simulink model "Electrical787"  (R2013a)
settings: Solver=ode45  StartTime=0.0  StopTime=MSSN.gen.time(end)  RelTol=1e-3
InitFcn:
  | load('SampleOutput.mat')
  | 
  | load('SampleFuelBurn.mat')
undefined symbols (not defined in the file): ailerons, B_737, elevator, FuelBurn, landing_gear, rudder, thrust_rev
libraries: PowerFlowLib x95, simulink x17
(part 16 of 17)

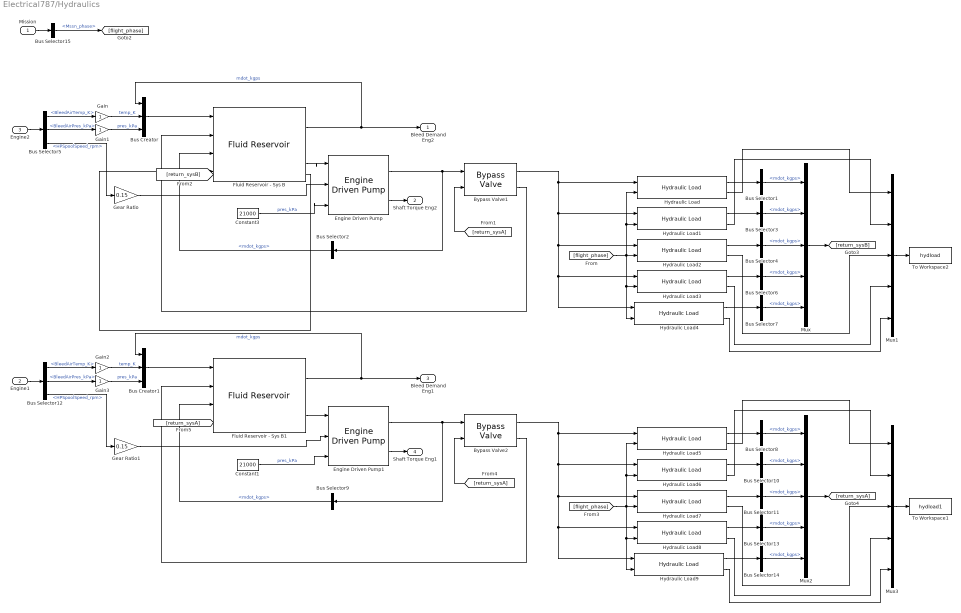
== system Electrical787/Hydraulics  ==
  Mission : Inport
  Engine1 : Inport  Port=2
  Engine2 : Inport  Port=3
  Bus Creator : BusCreator  Inputs=3
  Bus Creator1 : BusCreator  Inputs=3
  Bus Selector{1..4,6..11,13..14} (12 alike) : BusSelector  OutputSignals=mdot_kgps
  Bus Selector12 : BusSelector  OutputSignals=Bleed.BleedAirTemp_K,Bleed.BleedAirPres_kPa,Spools.HPSpoolSpeed_rpm
  Bus Selector15 : BusSelector  OutputSignals=Mssn_phase
  Bus Selector5 : BusSelector  OutputSignals=Bleed.BleedAirTemp_K,Bleed.BleedAirPres_kPa,Spools.HPSpoolSpeed_rpm
  Bypass Valve1 : PowerFlowLib/Energy & Power Systems/Hydraulic/Bypass Valve
  Bypass Valve2 : PowerFlowLib/Energy & Power Systems/Hydraulic/Bypass Valve
  Constant1 : Constant  Value=21000
  Constant3 : Constant  Value=21000
  Engine Driven Pump : PowerFlowLib/Energy & Power Systems/Hydraulic/Engine Driven Pump  RPM=3750  disp=39  eta_mech=95  eta_v=85  nom_T=40  nom_w=393  nom_delP=20684
  Engine Driven Pump1 : PowerFlowLib/Energy & Power Systems/Hydraulic/Engine Driven Pump  RPM=3750  disp=39  eta_mech=95  eta_v=85  nom_T=40  nom_w=393  nom_delP=20684
  Fluid Reservoir - Sys B : PowerFlowLib/Energy & Power Systems/Hydraulic/Fluid Reservoir  res_vol=.25  bleed_flowrate=.05  pres_loss=1  T_init=300  P_init=1500  mass_init=30
  Fluid Reservoir - Sys B1 : PowerFlowLib/Energy & Power Systems/Hydraulic/Fluid Reservoir  res_vol=.25  bleed_flowrate=.05  pres_loss=1  T_init=300  P_init=1500  mass_init=30
  Gain{,1..3} (4 alike) : Gain
  Gear Ratio : Gain  Gain=0.15
  Gear Ratio1 : Gain  Gain=0.15
  Hydraulic Load : PowerFlowLib/Energy & Power Systems/Hydraulic/Hydraulic Load  fileslct=off  filename=HydraulicLoad.mat  filedir=C:\Users\mwillms4\Dropbox\School\Graduate\Research\PowerFlow Development\PowerFlow Summer 2013\PropertyTables\HydraulicLoad.mat  var_struct=HydraulicLoad  h_load=B_737 - rudder
  Hydraulic Load1 : PowerFlowLib/Energy & Power Systems/Hydraulic/Hydraulic Load  fileslct=off  filename=HydraulicLoad.mat  filedir=C:\Users\mwillms4\Dropbox\School\Graduate\Research\PowerFlow Development\PowerFlow Summer 2013\PropertyTables\HydraulicLoad.mat  var_struct=HydraulicLoad  h_load=B_737 - ailerons
  Hydraulic Load2 : PowerFlowLib/Energy & Power Systems/Hydraulic/Hydraulic Load  fileslct=off  filename=HydraulicLoad.mat  filedir=C:\Users\mwillms4\Dropbox\School\Graduate\Research\PowerFlow Development\PowerFlow Summer 2013\PropertyTables\HydraulicLoad.mat  var_struct=HydraulicLoad  h_load=B_737 - elevator
  Hydraulic Load3 : PowerFlowLib/Energy & Power Systems/Hydraulic/Hydraulic Load  fileslct=off  filename=HydraulicLoad.mat  filedir=C:\Users\mwillms4\Dropbox\School\Graduate\Research\PowerFlow Development\PowerFlow Summer 2013\PropertyTables\HydraulicLoad.mat  var_struct=HydraulicLoad  h_load=B_737 - landing_gear
  Hydraulic Load4 : PowerFlowLib/Energy & Power Systems/Hydraulic/Hydraulic Load  fileslct=off  filename=HydraulicLoad.mat  filedir=C:\Users\mwillms4\Dropbox\School\Graduate\Research\PowerFlow Development\PowerFlow Summer 2013\PropertyTables\HydraulicLoad.mat  var_struct=HydraulicLoad  h_load=B_737 - thrust_rev
  Hydraulic Load5 : PowerFlowLib/Energy & Power Systems/Hydraulic/Hydraulic Load  fileslct=off  filename=HydraulicLoad.mat  filedir=C:\Users\mwillms4\Dropbox\School\Graduate\Research\PowerFlow Development\PowerFlow Summer 2013\PropertyTables\HydraulicLoad.mat  var_struct=HydraulicLoad  h_load=B_737 - rudder
  Hydraulic Load6 : PowerFlowLib/Energy & Power Systems/Hydraulic/Hydraulic Load  fileslct=off  filename=HydraulicLoad.mat  filedir=C:\Users\mwillms4\Dropbox\School\Graduate\Research\PowerFlow Development\PowerFlow Summer 2013\PropertyTables\HydraulicLoad.mat  var_struct=HydraulicLoad  h_load=B_737 - ailerons
  Hydraulic Load7 : PowerFlowLib/Energy & Power Systems/Hydraulic/Hydraulic Load  fileslct=off  filename=HydraulicLoad.mat  filedir=C:\Users\mwillms4\Dropbox\School\Graduate\Research\PowerFlow Development\PowerFlow Summer 2013\PropertyTables\HydraulicLoad.mat  var_struct=HydraulicLoad  h_load=B_737 - elevator
  Hydraulic Load8 : PowerFlowLib/Energy & Power Systems/Hydraulic/Hydraulic Load  fileslct=off  filename=HydraulicLoad.mat  filedir=C:\Users\mwillms4\Dropbox\School\Graduate\Research\PowerFlow Development\PowerFlow Summer 2013\PropertyTables\HydraulicLoad.mat  var_struct=HydraulicLoad  h_load=B_737 - landing_gear
  Hydraulic Load9 : PowerFlowLib/Energy & Power Systems/Hydraulic/Hydraulic Load  fileslct=off  filename=HydraulicLoad.mat  filedir=C:\Users\mwillms4\Dropbox\School\Graduate\Research\PowerFlow Development\PowerFlow Summer 2013\PropertyTables\HydraulicLoad.mat  var_struct=HydraulicLoad  h_load=B_737 - thrust_rev
  Mux{,1..3} (4 alike) : Mux  Inputs=5
  To Workspace1 : ToWorkspace  VariableName=hydload1  SampleTime=10  SaveFormat=Structure With Time
  To Workspace2 : ToWorkspace  VariableName=hydload  SampleTime=10  SaveFormat=Structure With Time
  Bleed Demand Eng2 : Outport
  Shaft Torque Eng2 : Outport  Port=2
  Bleed Demand Eng1 : Outport  Port=3
  Shaft Torque Eng1 : Outport  Port=4
  wires:
  Bus Creator/1 -> Fluid Reservoir - Sys B/1
  Bus Selector5/1 -> Gain/1  "<BleedAirTemp_K>"
  Bus Selector5/2 -> Gain1/1  "<BleedAirPres_kPa>"
  Hydraulic Load/1 -> Bus Selector1/1
  Fluid Reservoir - Sys B/2 -> Engine Driven Pump/1
  Engine Driven Pump/1 -> Bypass Valve1/1, Bus Selector2/1
  Bypass Valve1/1 -> Hydraulic Load3/1, Hydraulic Load4/1, Hydraulic Load2/1, Hydraulic Load1/1, Hydraulic Load/1
  Gear Ratio/1 -> Engine Driven Pump/2
  Bus Selector2/1 -> Fluid Reservoir - Sys B/3  "<mdot_kgps>"
  Bypass Valve1/2 -> Fluid Reservoir - Sys B/2
  Fluid Reservoir - Sys B/1 -> Bus Creator/1, Bleed Demand Eng2/1  "mdot_kgps"
  Hydraulic Load1/2 -> Mux1/2
  Hydraulic Load2/2 -> Mux1/3
  Hydraulic Load1/1 -> Bus Selector3/1
  Hydraulic Load2/1 -> Bus Selector4/1
  Bus Selector3/1 -> Mux/2  "<mdot_kgps>"
  Bus Selector1/1 -> Mux/1  "<mdot_kgps>"
  Bus Selector4/1 -> Mux/3  "<mdot_kgps>"
  Mux/1 -> [return_sysB]
  [return_sysA] -> Bypass Valve1/2
  [return_sysB] -> Fluid Reservoir - Sys B/4
  [flight_phase] -> Hydraulic Load/2, Hydraulic Load1/2, Hydraulic Load3/2, Hydraulic Load4/2, Hydraulic Load2/2
  Engine2/1 -> Bus Selector5/1
  Hydraulic Load3/1 -> Bus Selector6/1
  Hydraulic Load4/1 -> Bus Selector7/1
  Hydraulic Load4/2 -> Mux1/5
  Hydraulic Load3/2 -> Mux1/4
  Bus Selector6/1 -> Mux/4  "<mdot_kgps>"
  Bus Selector7/1 -> Mux/5  "<mdot_kgps>"
  Mission/1 -> Bus Selector15/1
  Bus Selector15/1 -> [flight_phase]  "<Mssn_phase>"
  Gain/1 -> Bus Creator/2  "temp_K"
  Gain1/1 -> Bus Creator/3  "pres_kPa"
  Constant3/1 -> Engine Driven Pump/3  "pres_kPa"
  Hydraulic Load/2 -> Mux1/1
  Bus Selector5/3 -> Gear Ratio/1  "<HPSpoolSpeed_rpm>"
  Engine Driven Pump/2 -> Shaft Torque Eng2/1
  Mux1/1 -> To Workspace2/1
  Bus Creator1/1 -> Fluid Reservoir - Sys B1/1
  Bus Selector12/1 -> Gain2/1  "<BleedAirTemp_K>"
  Bus Selector12/2 -> Gain3/1  "<BleedAirPres_kPa>"
  Hydraulic Load5/1 -> Bus Selector8/1
  Fluid Reservoir - Sys B1/2 -> Engine Driven Pump1/1
  Engine Driven Pump1/1 -> Bus Selector9/1, Bypass Valve2/1
  Bypass Valve2/1 -> Hydraulic Load8/1, Hydraulic Load9/1, Hydraulic Load7/1, Hydraulic Load6/1, Hydraulic Load5/1
  Gear Ratio1/1 -> Engine Driven Pump1/2
  Bus Selector9/1 -> Fluid Reservoir - Sys B1/3  "<mdot_kgps>"
  Bypass Valve2/2 -> Fluid Reservoir - Sys B1/2
  Fluid Reservoir - Sys B1/1 -> Bus Creator1/1, Bleed Demand Eng1/1  "mdot_kgps"
  Hydraulic Load6/2 -> Mux3/2
  Hydraulic Load7/2 -> Mux3/3
  Hydraulic Load6/1 -> Bus Selector10/1
  Hydraulic Load7/1 -> Bus Selector11/1
  Bus Selector10/1 -> Mux2/2  "<mdot_kgps>"
  Bus Selector8/1 -> Mux2/1  "<mdot_kgps>"
  Bus Selector11/1 -> Mux2/3  "<mdot_kgps>"
  Mux2/1 -> [return_sysA]
  [return_sysA] -> Bypass Valve2/2
  [return_sysA] -> Fluid Reservoir - Sys B1/4
  [flight_phase] -> Hydraulic Load5/2, Hydraulic Load6/2, Hydraulic Load8/2, Hydraulic Load9/2, Hydraulic Load7/2
  Engine1/1 -> Bus Selector12/1
  Hydraulic Load8/1 -> Bus Selector13/1
  Hydraulic Load9/1 -> Bus Selector14/1
  Hydraulic Load9/2 -> Mux3/5
  Hydraulic Load8/2 -> Mux3/4
  Bus Selector13/1 -> Mux2/4  "<mdot_kgps>"
  Bus Selector14/1 -> Mux2/5  "<mdot_kgps>"
  Gain2/1 -> Bus Creator1/2  "temp_K"
  Gain3/1 -> Bus Creator1/3  "pres_kPa"
  Constant1/1 -> Engine Driven Pump1/3  "pres_kPa"
  Hydraulic Load5/2 -> Mux3/1
  Bus Selector12/3 -> Gear Ratio1/1  "<HPSpoolSpeed_rpm>"
  Engine Driven Pump1/2 -> Shaft Torque Eng1/1
  Mux3/1 -> To Workspace1/1

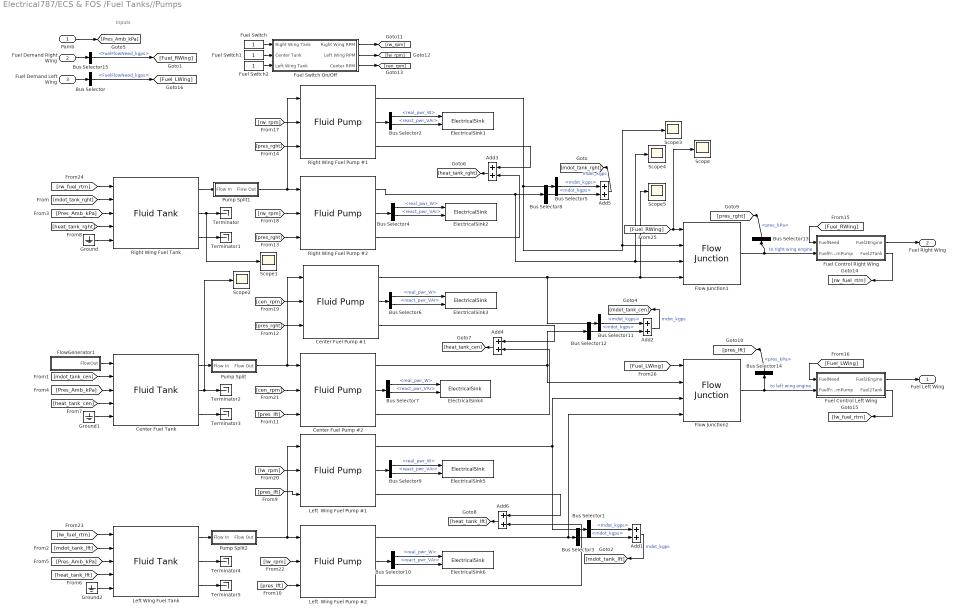
== system Electrical787/ECS & FOS /Fuel Tanks//Pumps ==
  note: Inputs
  Pamb : Inport
  Fuel Demand Right Wing : Inport  Port=2
  Fuel Demand Left Wing : Inport  Port=3
  Add{1..6} (6 alike) : Sum
  Bus Selector : BusSelector  OutputSignals=Fuel.FuelFlowNeed_kgps
  Bus Selector{1,3,5,8,11..12} (6 alike) : BusSelector  OutputSignals=mdot_kgps
  Bus Selector{2,4,6..7,9..10} (6 alike) : BusSelector  OutputSignals=real_pwr_W,react_pwr_VAr
  Bus Selector13 : BusSelector  OutputSignals=pres_kPa
  Bus Selector14 : BusSelector  OutputSignals=pres_kPa
  Bus Selector15 : BusSelector  OutputSignals=Fuel.FuelFlowNeed_kgps
  Center Fuel Pump #1 : PowerFlowLib/Energy & Power Systems/Thermal/Fuel & Oil/Fluid Pump  fld=Fuel  maptype=Pressure (kPa) vs. Vol. Flow Rate (m³/hr)  map=B737_AC_fuel1  map_load=off  SG=0.82  pump_eff=.75  heat_out=off  AC_pwr=on  pf=1  mech_pwr=off
  Center Fuel Pump #2 : PowerFlowLib/Energy & Power Systems/Thermal/Fuel & Oil/Fluid Pump  fld=Fuel  maptype=Pressure (kPa) vs. Vol. Flow Rate (m³/hr)  map=B737_AC_fuel1  map_load=off  SG=0.82  pump_eff=.75  heat_out=off  AC_pwr=on  pf=1  mech_pwr=off
  Center Fuel Tank : PowerFlowLib/Energy & Power Systems/Thermal/Fuel & Oil/Fluid Tank  fld=Fuel  fileslct=off  filename=fueltank_area.m  filedir=fueltank_area.m  tank_loc=Left Wing Tank  areaprompt2=off  max_vol=3.2  m_init=2500  fld_Tint=0  ull_Tint=30  Pover=100  HTC_fg=14.2  wallHXF=off  wetHTC=14.2  dryHTC=14.2  Qinternal=0
  ElectricalSink1 : PowerFlowLib/Support Functions//Tools/ElectricalSink  Tag=Flow  Description=TwoPhase  load_loc=RightWing  ACDC_load=AC  units=Watts  unq_id=9219
  ElectricalSink2 : PowerFlowLib/Support Functions//Tools/ElectricalSink  Tag=Flow  Description=TwoPhase  load_loc=RightWing  ACDC_load=AC  units=Watts  unq_id=5921
  ElectricalSink3 : PowerFlowLib/Support Functions//Tools/ElectricalSink  Tag=Flow  Description=TwoPhase  load_loc=RightWing  ACDC_load=AC  units=Watts  unq_id=9683
  ElectricalSink4 : PowerFlowLib/Support Functions//Tools/ElectricalSink  Tag=Flow  Description=TwoPhase  load_loc=LeftWing  ACDC_load=AC  units=Watts  unq_id=2143
  ElectricalSink5 : PowerFlowLib/Support Functions//Tools/ElectricalSink  Tag=Flow  Description=TwoPhase  load_loc=LeftWing  ACDC_load=AC  units=Watts  unq_id=2418
  ElectricalSink6 : PowerFlowLib/Support Functions//Tools/ElectricalSink  Tag=Flow  Description=TwoPhase  load_loc=LeftWing  ACDC_load=AC  units=Watts  unq_id=9734
  Flow Junction1 : PowerFlowLib/Energy & Power Systems/Thermal/Fuel & Oil/Flow Junction  Description=TwoPhase  fld=Fuel  V=.05  Bm=10^5  initPres=6000  initTemp=30
  Flow Junction2 : PowerFlowLib/Energy & Power Systems/Thermal/Fuel & Oil/Flow Junction  Description=TwoPhase  fld=Fuel  V=.05  Bm=10^5  initPres=6000  initTemp=30
  FlowGenerator1 : Subsystem  Tag=Flow  Description=TwoPhase  mask{fld_type1=null, flowrate=0, flowtemp=0, flowpres=00, flowenthalpy=0}
      mask prompts: fld_type1 "Fluid Type"; flowrate "Fluid Flow Rate (kg/s)"; flowtemp "Fluid Flow Temperature (C)"; flowpres "Fluid Flow Pressure (kPa)"; flowenthalpy "Fluid Flow Enthalpy (kJ/kg)"
      mask TypeOptions fld_type1: null
      mask Display: text(.5,.5,'Flow Source','horizontalAlignment','center','texmode','on')
  Fuel Control Left Wing : Subsystem
      mask Display:
      | port_label('input',1,'{\bf Fuel Need}','TexMode','on')
      | port_label('input',2,'{\bf Fuel In}','TexMode','on')
      | 
      | 
      | port_label('output',1,'{\bf Fuel to Eng.}','TexMode','on')
      | port_label('output',2,'{\bf Fuel Return}','TexMode','on')
  "Fuel Control Right Wing " : Subsystem
      mask Display:
      | port_label('input',1,'{\bf Fuel Need}','TexMode','on')
      | port_label('input',2,'{\bf Fuel In}','TexMode','on')
      | 
      | 
      | port_label('output',1,'{\bf Fuel to Eng.}','TexMode','on')
      | port_label('output',2,'{\bf Fuel Return}','TexMode','on')
  Fuel Switch : Constant
  Fuel Switch On/Off : Subsystem
  Fuel Switch1 : Constant
  Fuel Switch2 : Constant
  Ground : Ground
  Ground1 : Ground
  Ground2 : Ground
  Left  Wing Fuel Pump #1 : PowerFlowLib/Energy & Power Systems/Thermal/Fuel & Oil/Fluid Pump  fld=Fuel  maptype=Pressure (kPa) vs. Vol. Flow Rate (m³/hr)  map=B737_AC_fuel1  map_load=off  SG=0.82  pump_eff=.75  heat_out=off  AC_pwr=on  pf=1  mech_pwr=off
  Left  Wing Fuel Pump #2 : PowerFlowLib/Energy & Power Systems/Thermal/Fuel & Oil/Fluid Pump  fld=Fuel  maptype=Pressure (kPa) vs. Vol. Flow Rate (m³/hr)  map=B737_AC_fuel1  map_load=off  SG=0.82  pump_eff=.75  heat_out=off  AC_pwr=on  pf=1  mech_pwr=off
  Left Wing Fuel Tank : PowerFlowLib/Energy & Power Systems/Thermal/Fuel & Oil/Fluid Tank  fld=Fuel  fileslct=off  filename=fueltank_area.m  filedir=fueltank_area.m  tank_loc=Left Wing Tank  areaprompt2=off  max_vol=3.2  m_init=2500  fld_Tint=0  ull_Tint=30  Pover=100  HTC_fg=14.2  wallHXF=off  wetHTC=14.2  dryHTC=14.2  Qinternal=0
  Pump Split : Subsystem
  Pump Split1 : Subsystem
  Pump Split2 : Subsystem
  Right Wing Fuel Pump #1 : PowerFlowLib/Energy & Power Systems/Thermal/Fuel & Oil/Fluid Pump  fld=Fuel  maptype=Pressure (kPa) vs. Vol. Flow Rate (m³/hr)  map=B737_AC_fuel1  map_load=off  SG=0.82  pump_eff=.75  heat_out=off  AC_pwr=on  pf=1  mech_pwr=off
  Right Wing Fuel Pump #2 : PowerFlowLib/Energy & Power Systems/Thermal/Fuel & Oil/Fluid Pump  fld=Fuel  maptype=Pressure (kPa) vs. Vol. Flow Rate (m³/hr)  map=B737_AC_fuel1  map_load=off  SG=0.82  pump_eff=.75  heat_out=off  AC_pwr=on  pf=1  mech_pwr=off
  Right Wing Fuel Tank : PowerFlowLib/Energy & Power Systems/Thermal/Fuel & Oil/Fluid Tank  fld=Fuel  fileslct=off  filename=fueltank_area.m  filedir=fueltank_area.m  tank_loc=Left Wing Tank  areaprompt2=off  max_vol=3.2  m_init=2500  fld_Tint=0  ull_Tint=30  Pover=100  HTC_fg=14.2  wallHXF=off  wetHTC=14.2  dryHTC=14.2  Qinternal=0
  Scope{,1..5} (6 alike) : Scope
      Scope settings: SaveName=ScopeData21
      Scope1 settings: YMin=2498.9  YMax=2498.9  SaveName=ScopeData23
      Scope2 settings: SaveName=ScopeData25
      Scope3 settings: SaveName=ScopeData27
      Scope4 settings: SaveName=ScopeData28
      Scope5 settings: SaveName=ScopeData29
  Terminator{,1..5} (6 alike) : Terminator
  Fuel Left Wing : Outport
  Fuel Right Wing : Outport  Port=2
  wires:
  Pamb/1 -> [Pres_Amb_kPa]
  Fuel Switch/1 -> Fuel Switch On/Off/1(Right Wing Tank)
  Fuel Switch1/1 -> Fuel Switch On/Off/2(Center Tank)
  Fuel Switch2/1 -> Fuel Switch On/Off/3(Left Wing Tank)
  Fuel Switch On/Off/1(Right Wing RPM) -> [rw_rpm]
  Fuel Switch On/Off/2(Left Wing RPM) -> [lw_rpm]
  Fuel Switch On/Off/3(Center RPM) -> [cen_rpm]
  Left  Wing Fuel Pump #2/1 -> Flow Junction2/4, Bus Selector3/1
  [lw_fuel_rtrn] -> Left Wing Fuel Tank/1
  Left  Wing Fuel Pump #2/2 -> Bus Selector10/1
  Left  Wing Fuel Pump #1/1 -> Flow Junction2/3, Bus Selector1/1
  Left  Wing Fuel Pump #1/2 -> Bus Selector9/1
  Center Fuel Pump #2/1 -> Flow Junction2/2, Bus Selector12/1
  FlowGenerator1/1(FlowOut) -> Center Fuel Tank/1
  Center Fuel Pump #2/2 -> Bus Selector7/1
  Flow Junction2/1 -> Bus Selector14/1, Fuel Control Left Wing/2(FuelFromPump)  "to left wing engine"
  Center Fuel Pump #1/1 -> Bus Selector11/1, Flow Junction1/4, Scope5/1
  Center Fuel Pump #1/2 -> Bus Selector6/1
  Flow Junction1/1 -> Bus Selector13/1, "Fuel Control Right Wing "/2(FuelFromPump)  "to right wing engine"
  Center Fuel Tank/1 -> Pump Split/1(Flow In)
  Right Wing Fuel Pump #2/1 -> Bus Selector8/1, Flow Junction1/3, Scope4/1
  [rw_fuel_rtrn] -> Right Wing Fuel Tank/1
  Right Wing Fuel Pump #2/2 -> Bus Selector4/1
  Right Wing Fuel Pump #1/1 -> Bus Selector5/1, Flow Junction1/2, Scope3/1
  [rw_rpm] -> Right Wing Fuel Pump #1/2
  Right Wing Fuel Tank/1 -> Pump Split1/1(Flow In)
  Pump Split1/1(Flow Out) -> Right Wing Fuel Pump #2/1, Right Wing Fuel Pump #1/1
  Bus Selector8/1 -> Add5/2  "<mdot_kgps>"
  [mdot_tank_rght] -> Right Wing Fuel Tank/2
  [mdot_tank_cen] -> Center Fuel Tank/2
  [mdot_tank_lft] -> Left Wing Fuel Tank/2
  Pump Split/1(Flow Out) -> Center Fuel Pump #1/1, Center Fuel Pump #2/1
  Left Wing Fuel Tank/1 -> Pump Split2/1(Flow In)
  Bus Selector5/1 -> Add5/1  "<mdot_kgps>"
  Add5/1 -> [mdot_tank_rght]  "mdot_kgps"
  Bus Selector3/1 -> Add1/2  "<mdot_kgps>"
  Bus Selector1/1 -> Add1/1  "<mdot_kgps>"
  Add1/1 -> [mdot_tank_lft]  "mdot_kgps"
  Bus Selector12/1 -> Add2/2  "<mdot_kgps>"
  Bus Selector11/1 -> Add2/1  "<mdot_kgps>"
  Add2/1 -> [mdot_tank_cen]  "mdot_kgps"
  [Pres_Amb_kPa] -> Right Wing Fuel Tank/3
  [Pres_Amb_kPa] -> Center Fuel Tank/3
  [Pres_Amb_kPa] -> Left Wing Fuel Tank/3
  Add6/1 -> [heat_tank_lft]
  [heat_tank_lft] -> Left Wing Fuel Tank/4
  [heat_tank_cen] -> Center Fuel Tank/4
  [heat_tank_rght] -> Right Wing Fuel Tank/4
  Bus Selector13/1 -> [pres_rght]  "<pres_kPa>"
  [rw_rpm] -> Right Wing Fuel Pump #2/2
  [cen_rpm] -> Center Fuel Pump #1/2
  [cen_rpm] -> Center Fuel Pump #2/2
  [lw_rpm] -> Left  Wing Fuel Pump #1/2
  [lw_rpm] -> Left  Wing Fuel Pump #2/2
  Bus Selector14/1 -> [pres_lft]  "<pres_kPa>"
  [pres_lft] -> Left  Wing Fuel Pump #1/3
  [pres_lft] -> Left  Wing Fuel Pump #2/3
  [pres_lft] -> Center Fuel Pump #2/3
  [pres_rght] -> Center Fuel Pump #1/3
  [pres_rght] -> Right Wing Fuel Pump #2/3
  [pres_rght] -> Right Wing Fuel Pump #1/3
  [Fuel_LWing] -> Flow Junction2/1
  [Fuel_RWing] -> Flow Junction1/1, Scope/1
  Right Wing Fuel Tank/2 -> Terminator/1, Scope1/1
  Right Wing Fuel Tank/3 -> Terminator1/1
  Center Fuel Tank/2 -> Terminator2/1, Scope2/1
  Center Fuel Tank/3 -> Terminator3/1
  Left Wing Fuel Tank/2 -> Terminator4/1
  Left Wing Fuel Tank/3 -> Terminator5/1
  Ground/1 -> Right Wing Fuel Tank/5
  Ground1/1 -> Center Fuel Tank/5
  Ground2/1 -> Left Wing Fuel Tank/5
  Fuel Demand Left Wing/1 -> Bus Selector/1
  [Fuel_RWing] -> "Fuel Control Right Wing "/1(FuelNeed)
  [Fuel_LWing] -> Fuel Control Left Wing/1(FuelNeed)
  Fuel Control Left Wing/2(Fuel2Tank) -> [lw_fuel_rtrn]
  "Fuel Control Right Wing "/2(Fuel2Tank) -> [rw_fuel_rtrn]
  "Fuel Control Right Wing "/1(Fuel2Engine) -> Fuel Right Wing/1
  Fuel Control Left Wing/1(Fuel2Engine) -> Fuel Left Wing/1
  Pump Split2/1(Flow Out) -> Left  Wing Fuel Pump #1/1, Left  Wing Fuel Pump #2/1
  Bus Selector/1 -> [Fuel_LWing]  "<FuelFlowNeed_kgps>"
  Fuel Demand Right Wing/1 -> Bus Selector15/1
  Bus Selector15/1 -> [Fuel_RWing]  "<FuelFlowNeed_kgps>"
  Bus Selector2/1 -> ElectricalSink1/1  "<real_pwr_W>"
  Add4/1 -> [heat_tank_cen]
  Add3/1 -> [heat_tank_rght]
  Right Wing Fuel Pump #1/2 -> Bus Selector2/1
  Bus Selector2/2 -> ElectricalSink1/2  "<react_pwr_VAr>"
  Bus Selector4/1 -> ElectricalSink2/1  "<real_pwr_W>"
  Bus Selector4/2 -> ElectricalSink2/2  "<react_pwr_VAr>"
  Bus Selector6/1 -> ElectricalSink3/1  "<real_pwr_W>"
  Bus Selector6/2 -> ElectricalSink3/2  "<react_pwr_VAr>"
  Bus Selector7/1 -> ElectricalSink4/1  "<real_pwr_W>"
  Bus Selector7/2 -> ElectricalSink4/2  "<react_pwr_VAr>"
  Bus Selector9/1 -> ElectricalSink5/1  "<real_pwr_W>"
  Bus Selector9/2 -> ElectricalSink5/2  "<react_pwr_VAr>"
  Bus Selector10/1 -> ElectricalSink6/1  "<real_pwr_W>"
  Bus Selector10/2 -> ElectricalSink6/2  "<react_pwr_VAr>"
  Right Wing Fuel Pump #1/3 -> Add3/1
  Right Wing Fuel Pump #2/3 -> Add3/2
  Center Fuel Pump #1/3 -> Add4/1
  Center Fuel Pump #2/3 -> Add4/2
  Left  Wing Fuel Pump #1/3 -> Add6/1
  Left  Wing Fuel Pump #2/3 -> Add6/2

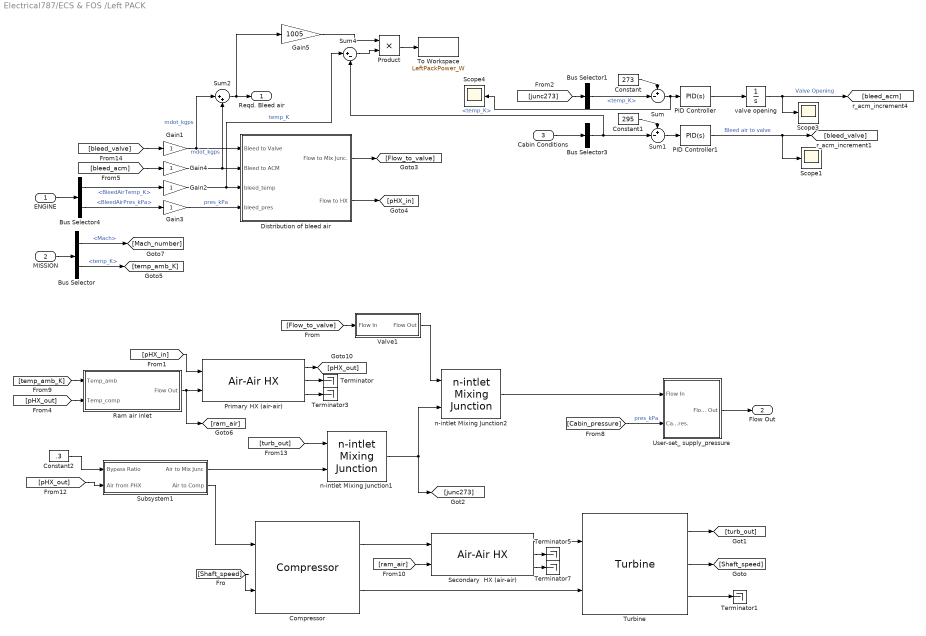
== system Electrical787/ECS & FOS /Left PACK ==
  ENGINE : Inport
  MISSION : Inport  Port=2
  Cabin Conditions : Inport  Port=3
  Bus Selector : BusSelector  OutputSignals=Flight parameters.Mach,Flight parameters.temp_K
  Bus Selector1 : BusSelector  OutputSignals=temp_K
  Bus Selector3 : BusSelector  OutputSignals=temp_K
  Bus Selector4 : BusSelector  OutputSignals=Bleed.BleedAirTemp_K,Bleed.BleedAirPres_kPa
  Compressor : PowerFlowLib/Energy & Power Systems/Thermal/ECS/Compressor
  Constant : Constant  Value=273
  Constant1 : Constant  Value=295
  Constant2 : Constant  Value=.3
  Distribution of bleed air : Subsystem
      mask Display:
      | port_label('input',1,'{ \bfBleed air to valve [kg/s]}','texmode','on')
      | port_label('input',2,'{ \bfBleed air to ACM [kg/s]}','texmode','on')
      | port_label('input',3,'{ \bfBleed temp. (K)}','texmode','on');
      | port_label('input',4,'{ \bfBleed pressure. (kPa)}','texmode','on')
      | 
      | 
      | 
      | port_label('output',1,'{\bfFlow to Mix Junc. }','texmode','on')
      | port_label('output',2,'{\bfFlow to ACM }','texmode','on')
  Gain{1..4} (4 alike) : Gain
  Gain5 : Gain  Gain=1005
  PID Controller : simulink/Continuous/PID Controller  Controller=PID  TimeDomain=Continuous-time  SampleTime=1  IntegratorMethod=Forward Euler  FilterMethod=Forward Euler  Form=Parallel  P=.01  I=0  D=0  N=100  InitialConditionSource=internal  InitialConditionForIntegrator=0  InitialConditionForFilter=0  ExternalReset=none  LimitOutput=off  UpperSaturationLimit=inf  LowerSaturationLimit=-inf  LinearizeAsGain=off  AntiWindupMode=none  Kb=1  TrackingMode=off  Kt=1  PParamMin=[]  PParamMax=[]  IParamMin=[]  IParamMax=[]  DParamMin=[]  DParamMax=[]  NParamMin=[]  NParamMax=[]  KbParamMin=[]  KbParamMax=[]  KtParamMin=[]  KtParamMax=[]  POutMin=[]  POutMax=[]  IOutMin=[]  IOutMax=[]  DOutMin=[]  DOutMax=[]  NOutMin=[]  NOutMax=[]  KbOutMin=[]  KbOutMax=[]  KtOutMin=[]  KtOutMax=[]  IntegratorOutMin=[]  IntegratorOutMax=[]  FilterOutMin=[]  FilterOutMax=[]  SumOutMin=[]  SumOutMax=[]  SumI1OutMin=[]  SumI1OutMax=[]  SumI2OutMin=[]  SumI2OutMax=[]  SumI3OutMin=[]  SumI3OutMax=[]  SumDOutMin=[]  SumDOutMax=[]  SaturationOutMin=[]  SaturationOutMax=[]  IntegratorContinuousStateAttributes=''  IntegratorStateMustResolveToSignalObject=off  IntegratorRTWStateStorageClass=Auto  FilterContinuousStateAttributes=''  FilterStateMustResolveToSignalObject=off  FilterRTWStateStorageClass=Auto
  PID Controller1 : simulink/Continuous/PID Controller  Controller=PID  TimeDomain=Continuous-time  SampleTime=1  IntegratorMethod=Forward Euler  FilterMethod=Forward Euler  Form=Parallel  P=.2  I=.01  D=0  N=100  InitialConditionSource=internal  InitialConditionForIntegrator=0  InitialConditionForFilter=0  ExternalReset=none  LimitOutput=on  UpperSaturationLimit=2  LowerSaturationLimit=.05  LinearizeAsGain=off  AntiWindupMode=clamping  Kb=1  TrackingMode=off  Kt=1  PParamMin=[]  PParamMax=[]  IParamMin=[]  IParamMax=[]  DParamMin=[]  DParamMax=[]  NParamMin=[]  NParamMax=[]  KbParamMin=[]  KbParamMax=[]  KtParamMin=[]  KtParamMax=[]  POutMin=[]  POutMax=[]  IOutMin=[]  IOutMax=[]  DOutMin=[]  DOutMax=[]  NOutMin=[]  NOutMax=[]  KbOutMin=[]  KbOutMax=[]  KtOutMin=[]  KtOutMax=[]  IntegratorOutMin=[]  IntegratorOutMax=[]  FilterOutMin=[]  FilterOutMax=[]  SumOutMin=[]  SumOutMax=[]  SumI1OutMin=[]  SumI1OutMax=[]  SumI2OutMin=[]  SumI2OutMax=[]  SumI3OutMin=[]  SumI3OutMax=[]  SumDOutMin=[]  SumDOutMax=[]  SaturationOutMin=[]  SaturationOutMax=[]  IntegratorContinuousStateAttributes=''  IntegratorStateMustResolveToSignalObject=off  IntegratorRTWStateStorageClass=Auto  FilterContinuousStateAttributes=''  FilterStateMustResolveToSignalObject=off  FilterRTWStateStorageClass=Auto
  Primary HX (air-air) : PowerFlowLib/Energy & Power Systems/Thermal/ECS/Air-Air HX  L_hx=0.2  W_hx=0.2  H_hx=0.2  t_p=0.0008  K_p=167  cp_hx=883  m_cm=16  l_fin=.005  t_fin=0.0002  s_fin=0.0015  h_fin=0.0095  K_n=167  eta_f=0.8  T_cm_0=50
  Product : Product
  Ram air inlet : Subsystem  mask{ram_air=.5, T_35=273}
      mask prompts: ram_air "Ram air mass flow rate"; T_35 "Temperature control for 35F valve"
      mask Display:
      | port_label('input',1,'{ \bf Ambient Temp.}','texmode','on')
      | port_label('input',2,'{ \bf Comp. Face Temp.}','texmode','on');
      | 
      | port_label('output',1,'{\bf Flow Out}','texmode','on')
  Scope1 : Scope
      settings: YMin=0.910804  YMax=0.910804  SaveName=ScopeData33  SampleInput=on  SampleTime=1
  Scope3 : Scope
      settings: YMin=0.738939  YMax=0.738939  SaveName=ScopeData35  SampleInput=on  SampleTime=1
  Scope4 : Scope
      settings: TimeRange=1500  YMin=2.8421709427e-013  YMax=2.8421709434e-013  SaveName=ScopeData37  SampleInput=on  SampleTime=1
  Secondary  HX (air-air) : PowerFlowLib/Energy & Power Systems/Thermal/ECS/Air-Air HX  L_hx=0.2  W_hx=0.2  H_hx=0.2  t_p=0.0008  K_p=167  cp_hx=883  m_cm=16  l_fin=.005  t_fin=0.0002  s_fin=0.0015  h_fin=0.0095  K_n=167  eta_f=0.8  T_cm_0=25
  Subsystem1 : Subsystem
  Sum : Sum  Inputs=+-|
  Sum1 : Sum  Inputs=+-|
  Sum2 : Sum  Inputs=|++
  Sum4 : Sum  Inputs=|+-
  Terminator{,1,3,5,7} (5 alike) : Terminator
  To Workspace : ToWorkspace  VariableName=LeftPackPower_W  SampleTime=10  SaveFormat=Structure With Time
  Turbine : PowerFlowLib/Energy & Power Systems/Thermal/ECS/Turbine  press_Turbine_exit=80  inertia=5e-5  n_t=0.7
  User-set_ supply_pressure : Subsystem
  Valve1 : Subsystem
  n-intlet Mixing Junction1 : PowerFlowLib/Energy & Power Systems/Thermal/ECS/n-intlet Mixing Junction  no_inlets=2  d_in_1=0.1  d_in_2=0.1  d_out=0.2
  n-intlet Mixing Junction2 : PowerFlowLib/Energy & Power Systems/Thermal/ECS/n-intlet Mixing Junction  no_inlets=2  d_in_1=0.1  d_in_2=0.1  d_out=0.2
  valve opening : Integrator  InitialCondition=.4  LimitOutput=on  UpperSaturationLimit=.8  LowerSaturationLimit=.2
  Reqd. Bleed air : Outport
  Flow Out : Outport  Port=2
  wires:
  Constant1/1 -> Sum1/1
  PID Controller1/1 -> [bleed_valve], Scope1/1  "Bleed air to valve"
  Sum1/1 -> PID Controller1/1
  Bus Selector3/1 -> Sum4/2, Sum1/2  "<temp_K>"
  [pHX_in] -> Primary HX (air-air)/1
  Valve1/1(Flow Out) -> n-intlet Mixing Junction2/1
  [Flow_to_valve] -> Valve1/1(Flow In)
  [Shaft_speed] -> Compressor/2
  Compressor/2 -> Turbine/2
  Ram air inlet/1(Flow Out) -> Primary HX (air-air)/2, [ram_air]
  Compressor/1 -> Secondary  HX (air-air)/1
  [ram_air] -> Secondary  HX (air-air)/2
  n-intlet Mixing Junction2/1 -> User-set_ supply_pressure/1(Flow In)
  Turbine/2 -> [Shaft_speed]
  Turbine/3 -> Terminator1/1
  Turbine/1 -> [turb_out]
  User-set_ supply_pressure/1(Flow Out) -> Flow Out/1
  [Cabin_pressure] -> User-set_ supply_pressure/2(Cabin Pres.)  "pres_kPa"
  [temp_amb_K] -> Ram air inlet/1(Temp_amb)
  [pHX_out] -> Ram air inlet/2(Temp_comp)
  MISSION/1 -> Bus Selector/1
  ENGINE/1 -> Bus Selector4/1
  Distribution of bleed air/2(Flow to HX) -> [pHX_in]
  Distribution of bleed air/1(Flow to Mix Junc.) -> [Flow_to_valve]
  Bus Selector4/1 -> Gain2/1  "<BleedAirTemp_K>"
  Bus Selector4/2 -> Gain3/1  "<BleedAirPres_kPa>"
  Bus Selector/2 -> [temp_amb_K]  "<temp_K>"
  Bus Selector/1 -> [Mach_number]  "<Mach>"
  Gain1/1 -> Distribution of bleed air/1(Bleed to Valve), Sum2/1  "mdot_kgps"
  Gain2/1 -> Sum4/1, Distribution of bleed air/3(bleed_temp)  "temp_K"
  Gain3/1 -> Distribution of bleed air/4(bleed_pres)  "pres_kPa"
  [bleed_valve] -> Gain1/1
  Primary HX (air-air)/3 -> Terminator3/1
  Primary HX (air-air)/2 -> Terminator/1
  Primary HX (air-air)/1 -> [pHX_out]
  Secondary  HX (air-air)/2 -> Terminator5/1
  Secondary  HX (air-air)/3 -> Terminator7/1
  Secondary  HX (air-air)/1 -> Turbine/1
  [pHX_out] -> Subsystem1/2(Air from PHX)
  n-intlet Mixing Junction1/1 -> n-intlet Mixing Junction2/2, [junc273]
  [turb_out] -> n-intlet Mixing Junction1/1
  Subsystem1/1(Air to Mix Junc) -> n-intlet Mixing Junction1/2
  Subsystem1/2(Air to Comp) -> Compressor/1
  [junc273] -> Bus Selector1/1
  Bus Selector1/1 -> Sum/2  "<temp_K>"
  Sum/1 -> PID Controller/1, Scope4/1
  PID Controller/1 -> valve opening/1
  valve opening/1 -> Scope3/1, [bleed_acm]  "Valve Opening"
  Constant/1 -> Sum/1
  Gain4/1 -> Distribution of bleed air/2(Bleed to ACM), Sum2/2  "mdot_kgps"
  Sum2/1 -> Gain5/1, Reqd. Bleed air/1
  Cabin Conditions/1 -> Bus Selector3/1
  [bleed_acm] -> Gain4/1
  Constant2/1 -> Subsystem1/1(Bypass Ratio)
  Gain5/1 -> Product/1
  Sum4/1 -> Product/2
  Product/1 -> To Workspace/1

== system Electrical787/ECS & FOS /Oil Tanks//Pumps Left Wing ==
  Oil Sys Pres : Inport
  Flow In : Inport  Port=2
  Bus Selector1 : BusSelector  OutputSignals=Oil
  Bus Selector2 : BusSelector  OutputSignals=real_pwr_W,react_pwr_VAr
  Bus Selector5 : BusSelector  OutputSignals=mdot_kgps,pres_kPa
  ElectricalSink1 : PowerFlowLib/Support Functions//Tools/ElectricalSink  Tag=Flow  Description=TwoPhase  load_loc=LeftWing  ACDC_load=AC  units=Watts  unq_id=1878
  Fluid Pump : PowerFlowLib/Energy & Power Systems/Thermal/Fuel & Oil/Fluid Pump  fld=Fuel  maptype=Pressure (kPa) vs. Vol. Flow Rate (m³/hr)  map=B737_AC_oil1  map_load=off  SG=0.82  pump_eff=.75  heat_out=off  AC_pwr=on  pf=1  mech_pwr=off
  Fluid Tank : PowerFlowLib/Energy & Power Systems/Thermal/Fuel & Oil/Fluid Tank  fld=Fuel  fileslct=off  filename=oiltank_area.m  filedir=C:\Users\mwillms4\Documents\GitHub\PowerFlow\SupportFunctions\oiltank_area.m  tank_loc=Left Wing Tank  areaprompt2=off  max_vol=0.00757082  m_init=5.5  fld_Tint=20  ull_Tint=30  Pover=100  HTC_fg=14.2  wallHXF=off  wetHTC=14.2  dryHTC=14.2  Qinternal=0
  Fuel Switch2 : Constant  Value=1400
  Ground : Ground
  Ground1 : Ground
  Terminator : Terminator
  Terminator1 : Terminator
  Oil To HX : Outport
  wires:
  Bus Selector5/1 -> Fluid Tank/2  "<mdot_kgps>"
  Fuel Switch2/1 -> Fluid Pump/2
  Flow In/1 -> Bus Selector1/1
  Oil Sys Pres/1 -> Fluid Pump/3
  Ground1/1 -> Fluid Tank/3
  Fluid Pump/1 -> Oil To HX/1, Bus Selector5/1
  ? -> Fluid Tank/4
  Ground/1 -> Fluid Tank/5
  Fluid Tank/3 -> Terminator1/1
  Fluid Tank/2 -> Terminator/1
  Fluid Tank/1 -> Fluid Pump/1
  Bus Selector2/1 -> ElectricalSink1/1  "<real_pwr_W>"
  Bus Selector2/2 -> ElectricalSink1/2  "<react_pwr_VAr>"
  Fluid Pump/2 -> Bus Selector2/1
  Bus Selector1/1 -> Fluid Tank/1  "<Oil>"

== system Electrical787/ECS & FOS /Oil Tanks//Pumps Left Wing1 ==
  Oil Sys Pres : Inport
  Flow In : Inport  Port=2
  Bus Selector1 : BusSelector  OutputSignals=Oil
  Bus Selector2 : BusSelector  OutputSignals=real_pwr_W,react_pwr_VAr
  Bus Selector5 : BusSelector  OutputSignals=mdot_kgps,pres_kPa
  ElectricalSink1 : PowerFlowLib/Support Functions//Tools/ElectricalSink  Tag=Flow  Description=TwoPhase  load_loc=LeftWing  ACDC_load=AC  units=Watts  unq_id=8332
  Fluid Pump : PowerFlowLib/Energy & Power Systems/Thermal/Fuel & Oil/Fluid Pump  fld=Fuel  maptype=Pressure (kPa) vs. Vol. Flow Rate (m³/hr)  map=B737_AC_oil1  map_load=off  SG=0.82  pump_eff=.75  heat_out=off  AC_pwr=on  pf=1  mech_pwr=off
  Fluid Tank : PowerFlowLib/Energy & Power Systems/Thermal/Fuel & Oil/Fluid Tank  fld=Fuel  fileslct=off  filename=oiltank_area.m  filedir=C:\Users\mwillms4\Documents\GitHub\PowerFlow\SupportFunctions\oiltank_area.m  tank_loc=Right Wing Tank  areaprompt2=off  max_vol=0.00757082  m_init=5.5  fld_Tint=20  ull_Tint=30  Pover=100  HTC_fg=14.2  wallHXF=off  wetHTC=14.2  dryHTC=14.2  Qinternal=0
  Fuel Switch2 : Constant  Value=1400
  Ground : Ground
  Ground1 : Ground
  Terminator : Terminator
  Terminator1 : Terminator
  Oil To HX : Outport
  wires:
  Bus Selector1/1 -> Fluid Tank/1  "<Oil>"
  Fluid Pump/2 -> Bus Selector2/1
  Bus Selector2/2 -> ElectricalSink1/2  "<react_pwr_VAr>"
  Bus Selector2/1 -> ElectricalSink1/1  "<real_pwr_W>"
  Fluid Tank/1 -> Fluid Pump/1
  Fluid Tank/2 -> Terminator/1
  Fluid Tank/3 -> Terminator1/1
  Ground/1 -> Fluid Tank/5
  ? -> Fluid Tank/4
  Fluid Pump/1 -> Bus Selector5/1, Oil To HX/1
  Ground1/1 -> Fluid Tank/3
  Oil Sys Pres/1 -> Fluid Pump/3
  Flow In/1 -> Bus Selector1/1
  Fuel Switch2/1 -> Fluid Pump/2
  Bus Selector5/1 -> Fluid Tank/2  "<mdot_kgps>"

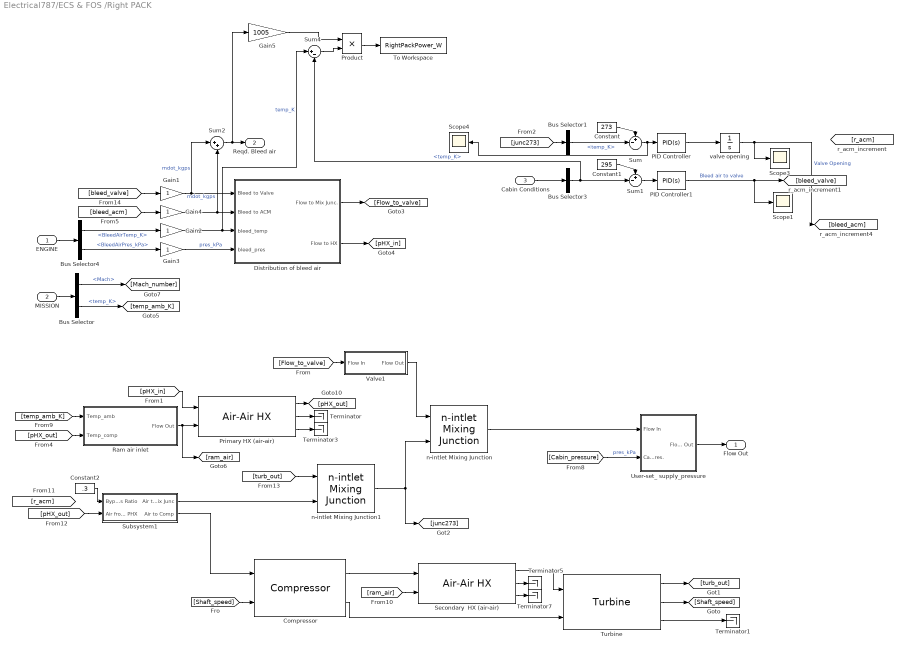
== system Electrical787/ECS & FOS /Right PACK ==
  ENGINE : Inport
  MISSION : Inport  Port=2
  Cabin Conditions : Inport  Port=3
  Bus Selector : BusSelector  OutputSignals=Flight parameters.Mach,Flight parameters.temp_K
  Bus Selector1 : BusSelector  OutputSignals=temp_K
  Bus Selector3 : BusSelector  OutputSignals=temp_K
  Bus Selector4 : BusSelector  OutputSignals=Bleed.BleedAirTemp_K,Bleed.BleedAirPres_kPa
  Compressor : PowerFlowLib/Energy & Power Systems/Thermal/ECS/Compressor
  Constant : Constant  Value=273
  Constant1 : Constant  Value=295
  Constant2 : Constant  Value=.3
  Distribution of bleed air : Subsystem
      mask Display:
      | port_label('input',1,'{ \bfBleed air to valve [kg/s]}','texmode','on')
      | port_label('input',2,'{ \bfBleed air to ACM [kg/s]}','texmode','on')
      | port_label('input',3,'{ \bfBleed temp. (K)}','texmode','on');
      | port_label('input',4,'{ \bfBleed pressure. (kPa)}','texmode','on')
      | 
      | 
      | 
      | port_label('output',1,'{\bfFlow to Mix Junc. }','texmode','on')
      | port_label('output',2,'{\bfFlow to ACM }','texmode','on')
  Gain{1..4} (4 alike) : Gain
  Gain5 : Gain  Gain=1005
  PID Controller : simulink/Continuous/PID Controller  Controller=PID  TimeDomain=Continuous-time  SampleTime=1  IntegratorMethod=Forward Euler  FilterMethod=Forward Euler  Form=Parallel  P=.01  I=0  D=0  N=100  InitialConditionSource=internal  InitialConditionForIntegrator=0  InitialConditionForFilter=0  ExternalReset=none  LimitOutput=off  UpperSaturationLimit=inf  LowerSaturationLimit=-inf  LinearizeAsGain=off  AntiWindupMode=none  Kb=1  TrackingMode=off  Kt=1  PParamMin=[]  PParamMax=[]  IParamMin=[]  IParamMax=[]  DParamMin=[]  DParamMax=[]  NParamMin=[]  NParamMax=[]  KbParamMin=[]  KbParamMax=[]  KtParamMin=[]  KtParamMax=[]  POutMin=[]  POutMax=[]  IOutMin=[]  IOutMax=[]  DOutMin=[]  DOutMax=[]  NOutMin=[]  NOutMax=[]  KbOutMin=[]  KbOutMax=[]  KtOutMin=[]  KtOutMax=[]  IntegratorOutMin=[]  IntegratorOutMax=[]  FilterOutMin=[]  FilterOutMax=[]  SumOutMin=[]  SumOutMax=[]  SumI1OutMin=[]  SumI1OutMax=[]  SumI2OutMin=[]  SumI2OutMax=[]  SumI3OutMin=[]  SumI3OutMax=[]  SumDOutMin=[]  SumDOutMax=[]  SaturationOutMin=[]  SaturationOutMax=[]  IntegratorContinuousStateAttributes=''  IntegratorStateMustResolveToSignalObject=off  IntegratorRTWStateStorageClass=Auto  FilterContinuousStateAttributes=''  FilterStateMustResolveToSignalObject=off  FilterRTWStateStorageClass=Auto
  PID Controller1 : simulink/Continuous/PID Controller  Controller=PID  TimeDomain=Continuous-time  SampleTime=1  IntegratorMethod=Forward Euler  FilterMethod=Forward Euler  Form=Parallel  P=.2  I=.01  D=0  N=100  InitialConditionSource=internal  InitialConditionForIntegrator=0  InitialConditionForFilter=0  ExternalReset=none  LimitOutput=on  UpperSaturationLimit=2  LowerSaturationLimit=.05  LinearizeAsGain=off  AntiWindupMode=clamping  Kb=1  TrackingMode=off  Kt=1  PParamMin=[]  PParamMax=[]  IParamMin=[]  IParamMax=[]  DParamMin=[]  DParamMax=[]  NParamMin=[]  NParamMax=[]  KbParamMin=[]  KbParamMax=[]  KtParamMin=[]  KtParamMax=[]  POutMin=[]  POutMax=[]  IOutMin=[]  IOutMax=[]  DOutMin=[]  DOutMax=[]  NOutMin=[]  NOutMax=[]  KbOutMin=[]  KbOutMax=[]  KtOutMin=[]  KtOutMax=[]  IntegratorOutMin=[]  IntegratorOutMax=[]  FilterOutMin=[]  FilterOutMax=[]  SumOutMin=[]  SumOutMax=[]  SumI1OutMin=[]  SumI1OutMax=[]  SumI2OutMin=[]  SumI2OutMax=[]  SumI3OutMin=[]  SumI3OutMax=[]  SumDOutMin=[]  SumDOutMax=[]  SaturationOutMin=[]  SaturationOutMax=[]  IntegratorContinuousStateAttributes=''  IntegratorStateMustResolveToSignalObject=off  IntegratorRTWStateStorageClass=Auto  FilterContinuousStateAttributes=''  FilterStateMustResolveToSignalObject=off  FilterRTWStateStorageClass=Auto
  Primary HX (air-air) : PowerFlowLib/Energy & Power Systems/Thermal/ECS/Air-Air HX  L_hx=0.2  W_hx=0.2  H_hx=0.2  t_p=0.0008  K_p=167  cp_hx=883  m_cm=16  l_fin=.005  t_fin=0.0002  s_fin=0.0015  h_fin=0.0095  K_n=167  eta_f=0.8  T_cm_0=50
  Product : Product
  Ram air inlet : Subsystem  mask{ram_air=.5, T_35=273}
      mask prompts: ram_air "Ram air mass flow rate"; T_35 "Temperature control for 35F valve"
      mask Display:
      | port_label('input',1,'{ \bf Ambient Temp.}','texmode','on')
      | port_label('input',2,'{ \bf Comp. Face Temp.}','texmode','on');
      | 
      | port_label('output',1,'{\bf Flow Out}','texmode','on')
  Scope1 : Scope
      settings: YMin=0  YMax=0.375  SaveName=ScopeData33  SampleInput=on  SampleTime=1
  Scope3 : Scope
      settings: YMin=0.427  YMax=0.437  SaveName=ScopeData35  SampleInput=on  SampleTime=1
  Scope4 : Scope
      settings: YMin=0.048825  YMax=0.04905  SaveName=ScopeData37  SampleInput=on  SampleTime=1
  Secondary  HX (air-air) : PowerFlowLib/Energy & Power Systems/Thermal/ECS/Air-Air HX  L_hx=0.2  W_hx=0.2  H_hx=0.2  t_p=0.0008  K_p=167  cp_hx=883  m_cm=16  l_fin=.005  t_fin=0.0002  s_fin=0.0015  h_fin=0.0095  K_n=167  eta_f=0.8  T_cm_0=25
  Subsystem1 : Subsystem
  Sum : Sum  Inputs=+-|
  Sum1 : Sum  Inputs=+-|
  Sum2 : Sum  Inputs=|++
  Sum4 : Sum  Inputs=|+-
  Terminator{,1,3,5,7} (5 alike) : Terminator
  To Workspace : ToWorkspace  VariableName=RightPackPower_W  SampleTime=10  SaveFormat=Structure With Time
  Turbine : PowerFlowLib/Energy & Power Systems/Thermal/ECS/Turbine  press_Turbine_exit=80  inertia=5e-5  n_t=0.7
  User-set_ supply_pressure : Subsystem
  Valve1 : Subsystem
  n-intlet Mixing Junction : PowerFlowLib/Energy & Power Systems/Thermal/ECS/n-intlet Mixing Junction  no_inlets=2  d_in_1=0.1  d_in_2=0.1  d_out=0.2
  n-intlet Mixing Junction1 : PowerFlowLib/Energy & Power Systems/Thermal/ECS/n-intlet Mixing Junction  no_inlets=2  d_in_1=0.1  d_in_2=0.1  d_out=0.2
  valve opening : Integrator  InitialCondition=.5  LimitOutput=on  UpperSaturationLimit=0.8  LowerSaturationLimit=0.2
  Flow Out : Outport
  Reqd. Bleed air : Outport  Port=2
  wires:
  Cabin Conditions/1 -> Bus Selector3/1
  Gain4/1 -> Sum2/2, Distribution of bleed air/2(Bleed to ACM)  "mdot_kgps"
  Constant/1 -> Sum/1
  valve opening/1 -> Scope3/1, [bleed_acm]  "Valve Opening"
  PID Controller/1 -> valve opening/1
  Sum/1 -> Scope4/1, PID Controller/1
  Bus Selector1/1 -> Sum/2  "<temp_K>"
  [junc273] -> Bus Selector1/1
  Subsystem1/2(Air to Comp) -> Compressor/1
  Subsystem1/1(Air to Mix Junc) -> n-intlet Mixing Junction1/2
  [turb_out] -> n-intlet Mixing Junction1/1
  n-intlet Mixing Junction1/1 -> n-intlet Mixing Junction/2, [junc273]
  [pHX_out] -> Subsystem1/2(Air from PHX)
  Secondary  HX (air-air)/1 -> Turbine/1
  Secondary  HX (air-air)/3 -> Terminator7/1
  Secondary  HX (air-air)/2 -> Terminator5/1
  Primary HX (air-air)/1 -> [pHX_out]
  Primary HX (air-air)/2 -> Terminator/1
  Primary HX (air-air)/3 -> Terminator3/1
  [bleed_valve] -> Gain1/1
  Gain3/1 -> Distribution of bleed air/4(bleed_pres)  "pres_kPa"
  Gain1/1 -> Sum2/1, Distribution of bleed air/1(Bleed to Valve)  "mdot_kgps"
  Bus Selector/1 -> [Mach_number]  "<Mach>"
  Bus Selector/2 -> [temp_amb_K]  "<temp_K>"
  Bus Selector4/2 -> Gain3/1  "<BleedAirPres_kPa>"
  Bus Selector4/1 -> Gain2/1  "<BleedAirTemp_K>"
  Distribution of bleed air/1(Flow to Mix Junc.) -> [Flow_to_valve]
  Distribution of bleed air/2(Flow to HX) -> [pHX_in]
  ENGINE/1 -> Bus Selector4/1
  MISSION/1 -> Bus Selector/1
  [pHX_out] -> Ram air inlet/2(Temp_comp)
  [temp_amb_K] -> Ram air inlet/1(Temp_amb)
  [Cabin_pressure] -> User-set_ supply_pressure/2(Cabin Pres.)  "pres_kPa"
  User-set_ supply_pressure/1(Flow Out) -> Flow Out/1
  Turbine/1 -> [turb_out]
  Turbine/3 -> Terminator1/1
  Turbine/2 -> [Shaft_speed]
  n-intlet Mixing Junction/1 -> User-set_ supply_pressure/1(Flow In)
  [ram_air] -> Secondary  HX (air-air)/2
  Compressor/1 -> Secondary  HX (air-air)/1
  Ram air inlet/1(Flow Out) -> [ram_air], Primary HX (air-air)/2
  Compressor/2 -> Turbine/2
  [Shaft_speed] -> Compressor/2
  [Flow_to_valve] -> Valve1/1(Flow In)
  Valve1/1(Flow Out) -> n-intlet Mixing Junction/1
  [pHX_in] -> Primary HX (air-air)/1
  Sum1/1 -> PID Controller1/1
  PID Controller1/1 -> Scope1/1, [bleed_valve]  "Bleed air to valve"
  Constant1/1 -> Sum1/1
  [bleed_acm] -> Gain4/1
  Constant2/1 -> Subsystem1/1(Bypass Ratio)
  Bus Selector3/1 -> Sum4/2, Sum1/2  "<temp_K>"
  Gain2/1 -> Sum4/1, Distribution of bleed air/3(bleed_temp)  "temp_K"
  Sum2/1 -> Gain5/1, Reqd. Bleed air/1
  Gain5/1 -> Product/1
  Sum4/1 -> Product/2
  Product/1 -> To Workspace/1

== system Electrical787/ECS & FOS /Thermal_sources_from Electrical_power_model1 ==
  Gain : Gain
  Terminator : Terminator
  Terminator1 : Terminator
  Terminator2 : Terminator
  ThermalSource : Subsystem  Tag=Flow  Description=TwoPhase  mask(Thermal Source){load_loc=Cockpit}
      mask prompts: load_loc "Location"
      mask help: Output of all thermal loads from the selected location. Loads are in Watts.
      mask init:
      | init_thermal_sourcesink(1)
      settings: CopyFcn=|
      | vals = get_param(gcb,'MaskValues');
      | set_param(gcb,'MaskValues',[vals(1);num2str(0)]);
      mask TypeOptions load_loc: Cockpit | Cabin | CargoBay | LeftWing | RightWing | Empennage
      mask Display:
      | text(.5,.7,'Thermal Source','horizontalAlignment','center','texmode','on')
      | text(.5,.4,get_param(gcb,'load_loc'),'horizontalAlignment','center','texmode','on')
  ThermalSource3 : Subsystem  Tag=Flow  Description=TwoPhase  mask(Thermal Source){load_loc=RightWing}
      mask prompts: load_loc "Location"
      mask help: Output of all thermal loads from the selected location. Loads are in Watts.
      mask init:
      | init_thermal_sourcesink(1)
      settings: CopyFcn=|
      | vals = get_param(gcb,'MaskValues');
      | set_param(gcb,'MaskValues',[vals(1);num2str(0)]);
      mask TypeOptions load_loc: Cockpit | Cabin | CargoBay | LeftWing | RightWing | Empennage
      mask Display:
      | text(.5,.7,'Thermal Source','horizontalAlignment','center','texmode','on')
      | text(.5,.4,get_param(gcb,'load_loc'),'horizontalAlignment','center','texmode','on')
  ThermalSource4 : Subsystem  Tag=Flow  Description=TwoPhase  mask(Thermal Source){load_loc=Empennage}
      mask prompts: load_loc "Location"
      mask help: Output of all thermal loads from the selected location. Loads are in Watts.
      mask init:
      | init_thermal_sourcesink(1)
      settings: CopyFcn=|
      | vals = get_param(gcb,'MaskValues');
      | set_param(gcb,'MaskValues',[vals(1);num2str(0)]);
      mask TypeOptions load_loc: Cockpit | Cabin | CargoBay | LeftWing | RightWing | Empennage
      mask Display:
      | text(.5,.7,'Thermal Source','horizontalAlignment','center','texmode','on')
      | text(.5,.4,get_param(gcb,'load_loc'),'horizontalAlignment','center','texmode','on')
  ThermalSource5 : Subsystem  Tag=Flow  Description=TwoPhase  mask(Thermal Source){load_loc=LeftWing}
      mask prompts: load_loc "Location"
      mask help: Output of all thermal loads from the selected location. Loads are in Watts.
      mask init:
      | init_thermal_sourcesink(1)
      settings: CopyFcn=|
      | vals = get_param(gcb,'MaskValues');
      | set_param(gcb,'MaskValues',[vals(1);num2str(0)]);
      mask TypeOptions load_loc: Cockpit | Cabin | CargoBay | LeftWing | RightWing | Empennage
      mask Display:
      | text(.5,.7,'Thermal Source','horizontalAlignment','center','texmode','on')
      | text(.5,.4,get_param(gcb,'load_loc'),'horizontalAlignment','center','texmode','on')
  Thermal Loads : Outport
  wires:
  ThermalSource/1(Load) -> Gain/1
  Gain/1 -> Thermal Loads/1
  ThermalSource3/1(Load) -> Terminator1/1
  ThermalSource4/1(Load) -> Terminator2/1
  ThermalSource5/1(Load) -> Terminator/1

== system Electrical787/ELECTRICAL SYS /230 Vac Distr ==
  note: Generator Bus 1
  note: Generator Bus 2
  Gen 1 : Inport
  Gen 2 : Inport  Port=2
  Gen 3 : Inport  Port=3
  Gen 4 : Inport  Port=4
  Gen 5 : Inport  Port=5
  Gen 6 : Inport  Port=6
  I_Bus : Inport  Port=7
  Gain : Gain  Gain=1/2
  Gen Bus w/ APU switch : PowerFlowLib/Energy & Power Systems/Electrical/Systems/Gen Bus w// APU switch  LOWVLIMIT=90  UPVLIMIT=250  bus_st=2
  Gen Bus w/ APU switch1 : PowerFlowLib/Energy & Power Systems/Electrical/Systems/Gen Bus w// APU switch  LOWVLIMIT=90  UPVLIMIT=250  bus_st=2
  Terminator : Terminator
  Terminator1 : Terminator
  Vbus1 : Outport
  Vbus2 : Outport  Port=2
  tag scope: i_APU1=global, i_APU2=global, i_GND1=global, i_GND2=global, i_MAIN1=global, i_MAIN2=global
  wires:
  Gen Bus w/ APU switch/3 -> [i_APU1]
  Gen Bus w/ APU switch/4 -> [i_GND1]
  [Gen_Bus1] -> Gen Bus w/ APU switch/1
  Gen Bus w/ APU switch/2 -> [i_MAIN1]
  Gen Bus w/ APU switch1/3 -> [i_APU2]
  Gen Bus w/ APU switch1/4 -> [i_GND2]
  Gen Bus w/ APU switch1/2 -> [i_MAIN2]
  [Gen_Bus2] -> Gen Bus w/ APU switch1/1
  Gen 1/1 -> Gen Bus w/ APU switch/2
  Gen 3/1 -> Gen Bus w/ APU switch1/2
  Gen 5/1 -> Gen Bus w/ APU switch/3
  Gen 6/1 -> Gen Bus w/ APU switch1/3
  Gen Bus w/ APU switch/1 -> Vbus1/1
  Gen Bus w/ APU switch1/1 -> Vbus2/1
  I_Bus/1 -> Gain/1
  Gain/1 -> Gen Bus w/ APU switch1/6, Gen Bus w/ APU switch/6
  Gen 2/1 -> Terminator/1
  Gen 4/1 -> Terminator1/1

== system Electrical787/ELECTRICAL SYS /Automatic Transformer Rectifier Unit ==
  Vin dqo : Inport
  Iout dqo : Inport  Port=2
  Constant : Constant  Value=[0.5 0.5 0.5]
  Demux : Demux  Outputs=3
  Demux1 : Demux  Outputs=3
  Memory12 : Memory
  Mux1 : Mux  Inputs=3
  Mux2 : Mux  Inputs=3
  Three Phase Full Bridge Practical : PowerFlowLib/Energy & Power Systems/Electrical/Rectifiers/Three Phase Full Bridge Practical  C=100e-6  Rc=1
  abc to qd0 : PowerFlowLib/Energy & Power Systems/Electrical/Coordinate Transformation/abc to qd0
  qd0 to abc : PowerFlowLib/Energy & Power Systems/Electrical/Coordinate Transformation/qd0 to abc
  three-phase full-bridge inverter1 : PowerFlowLib/Energy & Power Systems/Electrical/Inverters/three-phase  full-bridge  inverter1
  Vout dqo : Outport
  Iin : Outport  Port=2
  wires:
  Three Phase Full Bridge Practical/1 -> three-phase full-bridge inverter1/2
  Constant/1 -> three-phase full-bridge inverter1/1
  three-phase full-bridge inverter1/1 -> Demux/1
  Demux/1 -> abc to qd0/1
  Demux/2 -> abc to qd0/2
  Demux/3 -> abc to qd0/3
  abc to qd0/1 -> Mux1/1
  abc to qd0/2 -> Mux1/2
  abc to qd0/3 -> Mux1/3
  three-phase full-bridge inverter1/2 -> Memory12/1
  Memory12/1 -> Three Phase Full Bridge Practical/2
  Demux1/1 -> qd0 to abc/1
  Demux1/2 -> qd0 to abc/2
  Demux1/3 -> qd0 to abc/3
  qd0 to abc/1 -> Mux2/1
  qd0 to abc/2 -> Mux2/2
  qd0 to abc/3 -> Mux2/3
  Mux2/1 -> three-phase full-bridge inverter1/3
  Three Phase Full Bridge Practical/2 -> Iin/1
  Mux1/1 -> Vout dqo/1
  Iout dqo/1 -> Demux1/1
  Vin dqo/1 -> Three Phase Full Bridge Practical/1

== system Electrical787/ELECTRICAL SYS /Bus Controls ==
  Constant{1..5} (5 alike) : Constant
  Gen_Bus1 : Outport
  Gen_Bus2 : Outport  Port=2
  270V_DC_Bus : Outport  Port=3
  115V_AC_Bus : Outport  Port=4
  28V_DC_Bus : Outport  Port=5
  wires:
  Constant3/1 -> 28V_DC_Bus/1
  Constant5/1 -> 115V_AC_Bus/1
  Constant2/1 -> 270V_DC_Bus/1
  Constant4/1 -> Gen_Bus2/1
  Constant1/1 -> Gen_Bus1/1

== system Electrical787/ELECTRICAL SYS /DC Bus 1 ==
  Select : Inport
  VDC_1 : Inport  Port=2
  VDC_2 : Inport  Port=3
  Load current : Inport  Port=4
  Compare To Constant : simulink/Logic and Bit Operations/Compare To Constant  relop=<=  const=3.0  OutDataTypeStr=boolean
  Compare To Constant1 : simulink/Logic and Bit Operations/Compare To Constant  relop=<=  const=3.0  OutDataTypeStr=boolean
  Constant : Constant  Value=[0]
  Multiport Switch : MultiPortSwitch  Inputs=2
  Switch : Switch  Criteria=u2 ~= 0
  Switch1 : Switch  Criteria=u2 ~= 0
  Vbus : Outport
  IDC_1 : Outport  Port=2
  IDC_2 : Outport  Port=3
  wires:
  Load current/1 -> Switch1/1, Switch/1
  Multiport Switch/1 -> Vbus/1
  VDC_1/1 -> Multiport Switch/2
  VDC_2/1 -> Multiport Switch/3
  Select/1 -> Multiport Switch/1, Compare To Constant/1, Compare To Constant1/1
  Compare To Constant/1 -> Switch/2
  Compare To Constant1/1 -> Switch1/2
  Constant/1 -> Switch/3, Switch1/3
  Switch/1 -> IDC_1/1
  Switch1/1 -> IDC_2/1

== system Electrical787/ELECTRICAL SYS /DC Bus 3 ==
  Select : Inport
  VDC_1 : Inport  Port=2
  VDC_2 : Inport  Port=3
  Load current : Inport  Port=4
  Compare To Constant : simulink/Logic and Bit Operations/Compare To Constant  relop=<=  const=3.0  OutDataTypeStr=boolean
  Compare To Constant1 : simulink/Logic and Bit Operations/Compare To Constant  relop=<=  const=3.0  OutDataTypeStr=boolean
  Constant : Constant  Value=[0]
  Multiport Switch : MultiPortSwitch  Inputs=2
  Switch : Switch  Criteria=u2 ~= 0
  Switch1 : Switch  Criteria=u2 ~= 0
  Vbus : Outport
  IDC_1 : Outport  Port=2
  IDC_2 : Outport  Port=3
  wires:
  Load current/1 -> Switch1/1, Switch/1
  Multiport Switch/1 -> Vbus/1
  VDC_1/1 -> Multiport Switch/2
  VDC_2/1 -> Multiport Switch/3
  Select/1 -> Multiport Switch/1, Compare To Constant/1, Compare To Constant1/1
  Compare To Constant/1 -> Switch/2
  Compare To Constant1/1 -> Switch1/2
  Constant/1 -> Switch/3, Switch1/3
  Switch/1 -> IDC_1/1
  Switch1/1 -> IDC_2/1
